simulink model "sysgenDWT"  (Simulink 7.0)
settings: Solver=ode45  StartTime=0.0  StopTime=4096+1024+100  RelTol=1e-3
PreLoadFcn:
  | xlrequire('imageData.mat'); xlrequire('PreLoadFcn');
PostLoadFcn:
  | open_system('sysgenDWT/Processor/Memory Controller','force'); pause(0.50); open_system('sysgenDWT');pause(0.50); close_system('sysgenDWT/Processor/Memory Controller');pause(0.50); close_system('sysgenDWT/Processor');
StopFcn:
  | xlrequire('StopFcn');
values from neighbouring files (symbols this model uses):
  b1Init = sysgenDWT_imageData( stride + dither )    [sysgenDWT_PreLoadFcn.m]
  b2Init = sysgenDWT_imageData( stride + not(dither) )    [sysgenDWT_PreLoadFcn.m]
libraries: xbsIndex_r4 x214, dspindex x4, dspmtrx3 x4, dspsnks4 x3, xbsCopyrightNotice_r4 x1, dspsrcs4 x1
(part 2 of 3)

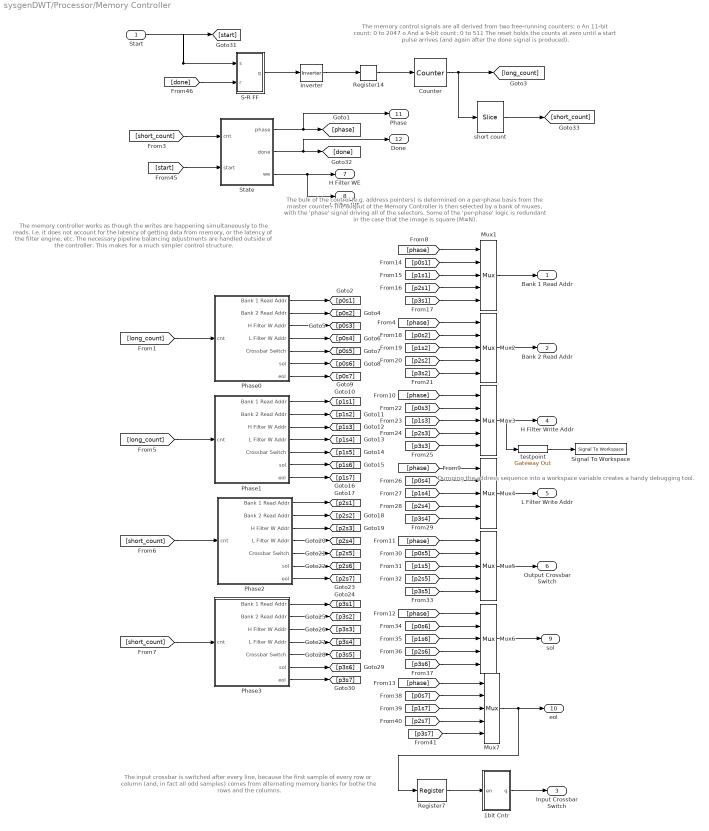
== system sysgenDWT/Processor/Memory Controller ==
  note: The memory control signals are all
      | derived from two free-running counters:
      |   o  An 11-bit count:    0 to 2047
      |   o  And a 9-bit count: 0 to 511
      | The reset holds the counts at zero until
      | a start pulse arrives (and again after the
      | done signal is produced).
  note: The bulk of the control (e.g. address pointers) is determined
      | on a per-phase basis from the master counter.  The output of
      | the Memory Controller is then selected by a bank of muxes,
      | with the 'phase' signal driving all of the selectors.  Some of
      | the 'per-phase' logic is redundant in the case that the image
      | is square (M=N).
  note: The memory controller works as though the
      | writes are happening simultaneously to the
      | reads. I.e. it does not account for the latency
      | of getting data from memory, or the latency
      | of the filter engine, etc.  The necessary
      | pipeline balancing adjustments are handled
      | outside of the controller.  This makes for a
      | much simpler control structure.
  note: The input crossbar is switched after every
      | line, because the first sample of every
      | row or column (and, in fact all odd samples)
      | comes from alternating memory banks for
      | bothe the rows and the columns.
  note: Dumping the address sequence
      | into a workspace variable creates
      | a handy debugging tool.
  Start : Inport  OutDataType=sfix(16)  OutScaling=2^0
  1bit Cntr : Subsystem
  Counter : xbsIndex_r4/Counter  cnt_type=Free Running  cnt_to=Inf  operation=Up  start_count=0  cnt_by_val=1  arith_type=Unsigned  n_bits=N+M-1  bin_pt=0  load_pin=off  rst=on  en=off  explicit_period=off  period=1  dbl_ovrd=off  use_behavioral_HDL=off  use_rpm=off  implementation=Fabric  block_type=counter
      settings: infoedit="Configurable up, down and up/down counter.<P><P>Hardware notes: Free running counters are the least expensive in hardware.  A count limited counter is implemented by combining a counter with a comparator."  xl_area=[6 11 0 11 0 0 0]  block_version=VER_STRING_GOES_HERE
  Inverter : xbsIndex_r4/Inverter  en=off  latency=0  dbl_ovrd=off  block_type=inv
      settings: xl_area=[1 0 0 1 0 0 0]  block_version=VER_STRING_GOES_HERE
  Mux{1..7} (7 alike) : xbsIndex_r4/Mux  inputs=4  en=off  latency=1  precision=Full  arith_type="Signed  (2's comp)"  n_bits=8  bin_pt=2  quantization=Truncate  overflow=Wrap  dbl_ovrd=off  block_type=mux
      Mux1 settings: xl_area=[11 11 0 22 0 0 0]  block_version=VER_STRING_GOES_HERE
      Mux2 settings: xl_area=[11 11 0 22 0 0 0]  block_version=VER_STRING_GOES_HERE
      Mux3 settings: xl_area=[11 11 0 22 0 0 0]  block_version=VER_STRING_GOES_HERE
      Mux4 settings: xl_area=[11 11 0 22 0 0 0]  block_version=VER_STRING_GOES_HERE
      Mux5 settings: xl_area=[1 1 0 2 0 0 0]  block_version=VER_STRING_GOES_HERE
      Mux6 settings: xl_area=[1 1 0 2 0 0 0]  block_version=VER_STRING_GOES_HERE
      Mux7 settings: xl_area=[1 1 0 2 0 0 0]  block_version=VER_STRING_GOES_HERE
  Phase0 : Subsystem
  Phase1 : Subsystem
  Phase2 : Subsystem
  Phase3 : Subsystem
  Register14 : xbsIndex_r4/Register  init=1  rst=off  en=off  dbl_ovrd=off  block_type=register
      settings: xl_area=[1 1 0 0 0 0 0]  block_version=VER_STRING_GOES_HERE
  Register7 : xbsIndex_r4/Register  init=0  rst=off  en=off  dbl_ovrd=off  block_type=register
      settings: xl_area=[1 1 0 0 0 0 0]  block_version=VER_STRING_GOES_HERE
  S-R FF : Subsystem
  Signal To Workspace : dspsnks4/Signal To Workspace  SystemSampleTime=-1  VariableName=HWriteAddr  FrameMode=Concatenate frames (2-D array)
      settings: FixptAsFi=off
  State : Subsystem
  short count : xbsIndex_r4/Slice  nbits=M+N-3  boolean_output=off  mode=Lower Bit Location + Width  bit1=0  base1=MSB of Input  bit0=0  base0=LSB of Input  dbl_ovrd=off  block_type=slice
      settings: infoedit="Extracts a given range of bits from each input sample and presents it at the output.  The output type is ordinarily unsigned with binary point at zero, but can be Boolean when the slice is one bit wide.<P><P>Hardware notes: In hardware this block costs nothing."  block_version=VER_STRING_GOES_HERE
  testpoint : xbsIndex_r4/Gateway Out  hdl_port=off  timing_constraint=None  locs_specified=off  LOCs={}  block_type=gatewayout
      settings: infoedit="Gateway out block.  Converts Xilinx fixed point inputs into ouputs of type Simulink integer, double, or fixed point.<P><P>Hardware notes:  In hardware these blocks become top level output ports or are discarded, depending on how they are configured."  xl_area=[0 0 0 0 0 0 0]  block_version=VER_STRING_GOES_HERE
  Bank 1 Read Addr : Outport  OutDataType=sfix(16)  OutScaling=2^0
  Bank 2 Read Addr : Outport  Port=2  OutDataType=sfix(16)  OutScaling=2^0
  Input Crossbar Switch : Outport  Port=3  OutDataType=sfix(16)  OutScaling=2^0
  H Filter Write Addr : Outport  Port=4  OutDataType=sfix(16)  OutScaling=2^0
  L Filter Write Addr : Outport  Port=5  OutDataType=sfix(16)  OutScaling=2^0
  Output Crossbar Switch : Outport  Port=6  OutDataType=sfix(16)  OutScaling=2^0
  H Filter WE : Outport  Port=7  OutDataType=sfix(16)  OutScaling=2^0
  L Filter WE : Outport  Port=8  OutDataType=sfix(16)  OutScaling=2^0
  sol : Outport  Port=9  OutDataType=sfix(16)  OutScaling=2^0
  eol : Outport  Port=10  OutDataType=sfix(16)  OutScaling=2^0
  Phase : Outport  Port=11  OutDataType=sfix(16)  OutScaling=2^0
  Done : Outport  Port=12  OutDataType=sfix(16)  OutScaling=2^0
  wires:
  Counter/1 -> [long_count], short count/1
  [long_count] -> Phase0/1(cnt)
  State/1(phase) -> Phase/1, [phase]
  [long_count] -> Phase1/1(cnt)
  [short_count] -> Phase2/1(cnt)
  [short_count] -> Phase3/1(cnt)
  [phase] -> Mux1/1
  [phase] -> Mux2/1
  [phase] -> Mux3/1
  [phase] -> Mux4/1
  [phase] -> Mux5/1
  [phase] -> Mux6/1
  [phase] -> Mux7/1
  Phase0/1(Bank 1 Read Addr) -> [p0s1]
  Phase0/2(Bank 2 Read Addr) -> [p0s2]
  Phase0/3(H Filter W Addr) -> [p0s3]
  Phase0/4(L Filter W Addr) -> [p0s4]
  Phase0/5(Crossbar Switch) -> [p0s5]
  Phase0/6(sol) -> [p0s6]
  Phase0/7(eol) -> [p0s7]
  Phase1/1(Bank 1 Read Addr) -> [p1s1]
  Phase1/2(Bank 2 Read Addr) -> [p1s2]
  Phase1/3(H Filter W Addr) -> [p1s3]
  Phase1/4(L Filter W Addr) -> [p1s4]
  Phase1/5(Crossbar Switch) -> [p1s5]
  Phase1/6(sol) -> [p1s6]
  Phase1/7(eol) -> [p1s7]
  Phase2/1(Bank 1 Read Addr) -> [p2s1]
  Phase2/2(Bank 2 Read Addr) -> [p2s2]
  Phase2/3(H Filter W Addr) -> [p2s3]
  Phase2/4(L Filter W Addr) -> [p2s4]
  Phase2/5(Crossbar Switch) -> [p2s5]
  Phase2/6(sol) -> [p2s6]
  Phase2/7(eol) -> [p2s7]
  Phase3/1(Bank 1 Read Addr) -> [p3s1]
  Phase3/2(Bank 2 Read Addr) -> [p3s2]
  Phase3/3(H Filter W Addr) -> [p3s3]
  Phase3/4(L Filter W Addr) -> [p3s4]
  Phase3/5(Crossbar Switch) -> [p3s5]
  Phase3/6(sol) -> [p3s6]
  Phase3/7(eol) -> [p3s7]
  [p0s1] -> Mux1/2
  [p1s1] -> Mux1/3
  [p2s1] -> Mux1/4
  [p3s1] -> Mux1/5
  [p0s2] -> Mux2/2
  [p1s2] -> Mux2/3
  [p2s2] -> Mux2/4
  [p3s2] -> Mux2/5
  [p0s3] -> Mux3/2
  [p1s3] -> Mux3/3
  [p2s3] -> Mux3/4
  [p3s3] -> Mux3/5
  [p0s4] -> Mux4/2
  [p1s4] -> Mux4/3
  [p2s4] -> Mux4/4
  [p3s4] -> Mux4/5
  [p0s5] -> Mux5/2
  [p1s5] -> Mux5/3
  [p2s5] -> Mux5/4
  [p3s5] -> Mux5/5
  [p0s6] -> Mux6/2
  [p1s6] -> Mux6/3
  [p2s6] -> Mux6/4
  [p3s6] -> Mux6/5
  [p0s7] -> Mux7/2
  [p1s7] -> Mux7/3
  [p2s7] -> Mux7/4
  [p3s7] -> Mux7/5
  Mux7/1 -> eol/1, Register7/1
  Mux6/1 -> sol/1
  Mux5/1 -> Output Crossbar Switch/1
  Mux4/1 -> L Filter Write Addr/1
  Mux3/1 -> H Filter Write Addr/1, testpoint/1
  Mux1/1 -> Bank 1 Read Addr/1
  Mux2/1 -> Bank 2 Read Addr/1
  1bit Cntr/1(q) -> Input Crossbar Switch/1
  Register7/1 -> 1bit Cntr/1(en)
  S-R FF/1(q) -> Inverter/1
  Start/1 -> S-R FF/1(s), [start]
  Register14/1 -> Counter/1
  Inverter/1 -> Register14/1
  [short_count] -> State/1(cnt)
  [start] -> State/2(start)
  State/3(we) -> L Filter WE/1, H Filter WE/1
  State/2(done) -> Done/1, [done]
  [done] -> S-R FF/2(r)
  short count/1 -> [short_count]
  testpoint/1 -> Signal To Workspace/1

== system sysgenDWT/Processor/Read Addr Crossbar ==
  note: Connect either A to A' and B to B'
      | or A to B' and B to A' based on
      | the signal "Cross".
  A : Inport  OutDataType=sfix(16)  OutScaling=2^0
  B : Inport  Port=2  OutDataType=sfix(16)  OutScaling=2^0
  Cross : Inport  Port=3  OutDataType=sfix(16)  OutScaling=2^0
  Mux2 : xbsIndex_r4/Mux  inputs=2  en=off  latency=0  precision=Full  arith_type="Signed  (2's comp)"  n_bits=8  bin_pt=2  quantization=Truncate  overflow=Wrap  dbl_ovrd=off  block_type=mux
      settings: xl_area=[6 0 0 11 0 0 0]  block_version=VER_STRING_GOES_HERE
  Mux3 : xbsIndex_r4/Mux  inputs=2  en=off  latency=0  precision=Full  arith_type="Signed  (2's comp)"  n_bits=8  bin_pt=2  quantization=Truncate  overflow=Wrap  dbl_ovrd=off  block_type=mux
      settings: xl_area=[6 0 0 11 0 0 0]  block_version=VER_STRING_GOES_HERE
  A' : Outport  OutDataType=sfix(16)  OutScaling=2^0
  B' : Outport  Port=2  OutDataType=sfix(16)  OutScaling=2^0
  wires:
  Cross/1 -> Mux3/1, Mux2/1
  B/1 -> Mux2/3, Mux3/2
  A/1 -> Mux3/3, Mux2/2
  Mux3/1 -> B'/1
  Mux2/1 -> A'/1

== system sysgenDWT/Processor/WE Crossbar ==
  note: Connect either A to A' and B to B'
      | or A to B' and B to A' based on
      | the signal "Cross".
  A : Inport  OutDataType=sfix(16)  OutScaling=2^0
  B : Inport  Port=2  OutDataType=sfix(16)  OutScaling=2^0
  Cross : Inport  Port=3  OutDataType=sfix(16)  OutScaling=2^0
  Mux2 : xbsIndex_r4/Mux  inputs=2  en=off  latency=1  precision=Full  arith_type="Signed  (2's comp)"  n_bits=8  bin_pt=2  quantization=Truncate  overflow=Wrap  dbl_ovrd=off  block_type=mux
      settings: xl_area=[1 1 0 1 0 0 0]  block_version=VER_STRING_GOES_HERE
  Mux3 : xbsIndex_r4/Mux  inputs=2  en=off  latency=1  precision=Full  arith_type="Signed  (2's comp)"  n_bits=8  bin_pt=2  quantization=Truncate  overflow=Wrap  dbl_ovrd=off  block_type=mux
      settings: xl_area=[1 1 0 1 0 0 0]  block_version=VER_STRING_GOES_HERE
  A' : Outport  OutDataType=sfix(16)  OutScaling=2^0
  B' : Outport  Port=2  OutDataType=sfix(16)  OutScaling=2^0
  wires:
  Mux2/1 -> A'/1
  Mux3/1 -> B'/1
  A/1 -> Mux2/2, Mux3/3
  B/1 -> Mux3/2, Mux2/3
  Cross/1 -> Mux2/1, Mux3/1

== system sysgenDWT/Processor/Write Addr Crossbar ==
  note: Connect either A to A' and B to B'
      | or A to B' and B to A' based on
      | the signal "Cross".
  A : Inport  OutDataType=sfix(16)  OutScaling=2^0
  B : Inport  Port=2  OutDataType=sfix(16)  OutScaling=2^0
  Cross : Inport  Port=3  OutDataType=sfix(16)  OutScaling=2^0
  Mux2 : xbsIndex_r4/Mux  inputs=2  en=off  latency=1  precision=Full  arith_type="Signed  (2's comp)"  n_bits=8  bin_pt=2  quantization=Truncate  overflow=Wrap  dbl_ovrd=off  block_type=mux
      settings: xl_area=[6 11 0 11 0 0 0]  block_version=VER_STRING_GOES_HERE
  Mux3 : xbsIndex_r4/Mux  inputs=2  en=off  latency=1  precision=Full  arith_type="Signed  (2's comp)"  n_bits=8  bin_pt=2  quantization=Truncate  overflow=Wrap  dbl_ovrd=off  block_type=mux
      settings: xl_area=[6 11 0 11 0 0 0]  block_version=VER_STRING_GOES_HERE
  A' : Outport  OutDataType=sfix(16)  OutScaling=2^0
  B' : Outport  Port=2  OutDataType=sfix(16)  OutScaling=2^0
  wires:
  Mux2/1 -> A'/1
  Mux3/1 -> B'/1
  A/1 -> Mux2/2, Mux3/3
  B/1 -> Mux3/2, Mux2/3
  Cross/1 -> Mux2/1, Mux3/1

== system sysgenDWT/Processor/Memory Controller/1bit Cntr ==
  note: A 1-bit, synchronous counter.
      |
      | The Convert block does no work, it
      | just gives simulink a hint as to what
      | the feedback type is.
  en : Inport  OutDataType=sfix(16)  OutScaling=2^0
  Convert : xbsIndex_r4/Convert  Orientation=left  arith_type=Unsigned  n_bits=1  bin_pt=0  quantization=Truncate  overflow=Wrap  latency=0  dbl_ovrd=off  pipeline=off  block_type=convert
      settings: infoedit=The input is presented at the output after quantization and overflow effects.<P><P>Hardware notes: Additional hardware is used when rounding or saturation is selected and output width is less than the input width.  xl_area=[0 0 0 0 0 0 0]  block_version=VER_STRING_GOES_HERE
  Inverter1 : xbsIndex_r4/Inverter  en=off  latency=0  dbl_ovrd=off  block_type=inv
      settings: xl_area=[1 0 0 1 0 0 0]  block_version=VER_STRING_GOES_HERE
  Register6 : xbsIndex_r4/Register  init=1  rst=off  en=on  dbl_ovrd=off  block_type=register
      settings: xl_area=[1 1 0 0 0 0 0]  block_version=VER_STRING_GOES_HERE
  q : Outport  OutDataType=sfix(16)  OutScaling=2^0
  wires:
  Inverter1/1 -> Register6/1
  Register6/1 -> Convert/1, q/1
  Convert/1 -> Inverter1/1
  en/1 -> Register6/2

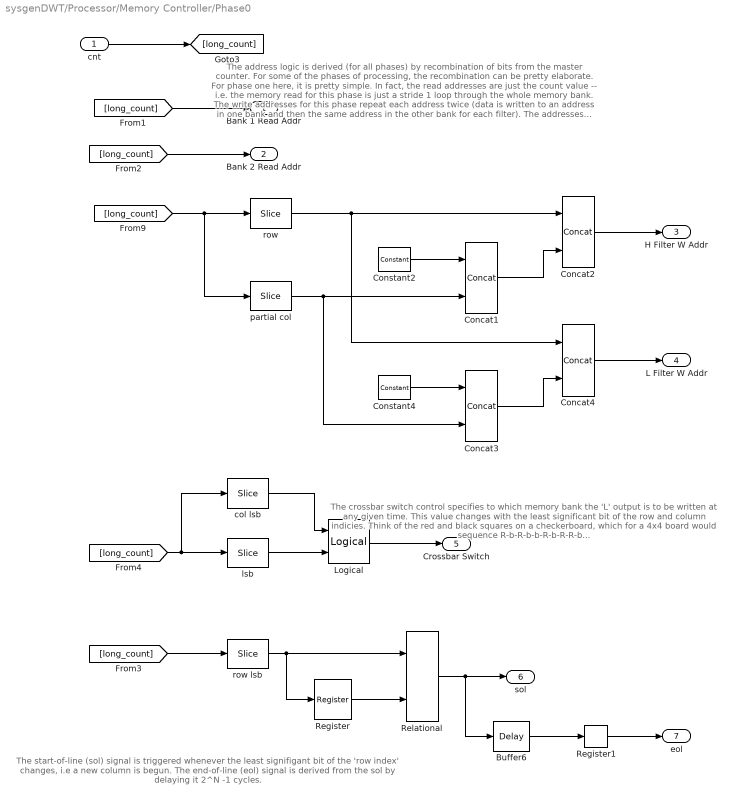
== system sysgenDWT/Processor/Memory Controller/Phase0 ==
  note: The address logic is derived (for all phases) by recombination
      | of bits from the master counter. For some of the phases of
      | processing, the recombination can be pretty elaborate.  For
      | phase one here, it is pretty simple.  In fact, the read addresses
      | are just the count value -- i.e. the memory read for this phase
      | is just a stride 1 loop through the whole memory bank.  The
      | write addresses for this phase repeat each address twice (data
      | is written to an address in one bank and then the same address
      | in the other bank for each filter).  The addresses increment by
      | one as each column is processed, and then jump to the next
      | column. A '1' is injected into the H address and a '0' into the 'L'
      | adress to write to the lower or upper half of memory, respectively.
  note: The crossbar switch control specifies to which memory
      | bank the 'L' output is to be written at any given time.
      | This value changes with the least significant bit of the
      | row and column indicies.  Think of the red and black
      | squares on a checkerboard, which for a 4x4 board would
      | sequence R-b-R-b-b-R-b-R-R-b...
  note: The start-of-line (sol) signal is triggered whenever the
      | least signifigant bit of the 'row index' changes, i.e a
      | new column is begun.  The end-of-line (eol) signal is
      | derived from the sol by delaying it 2^N -1 cycles.
  cnt : Inport  OutDataType=sfix(16)  OutScaling=2^0
  Buffer6 : xbsIndex_r4/Delay  en=off  latency=power(2,N-1)-2  dbl_ovrd=off  reg_retiming=off  block_type=delay
      settings: infoedit="Delay line having  configurable length.<P><P>Hardware notes: A delay line is a chain, each link of which is an SRL16 followed by a flip-flop. If register retiming is enabled, the delay line is a chain of flip-flops."  xl_area=[2 2 0 2 0 0 0]  block_version=VER_STRING_GOES_HERE
  Concat{1..4} (4 alike) : xbsIndex_r4/Concat  num_inputs=2  dbl_ovrd=off  block_type=concat
      settings: block_version=VER_STRING_GOES_HERE
  Constant2 : xbsIndex_r4/Constant  arith_type=Unsigned  const=1  n_bits=1  bin_pt=0  explicit_period=off  period=1  equ=P=C  opselect=C  inp2=PCIN>>17  opr=+  inp1=P  carry=CIN  dbl_ovrd=off  block_type=constant
      settings: block_version=VER_STRING_GOES_HERE
  Constant4 : xbsIndex_r4/Constant  arith_type=Unsigned  const=0  n_bits=1  bin_pt=0  explicit_period=off  period=1  equ=P=C  opselect=C  inp2=PCIN>>17  opr=+  inp1=P  carry=CIN  dbl_ovrd=off  block_type=constant
      settings: block_version=VER_STRING_GOES_HERE
  Logical : xbsIndex_r4/Logical  logical_function=XNOR  inputs=2  en=off  latency=0  precision=Full  arith_type=Unsigned  n_bits=8  bin_pt=2  align_bp=on  dbl_ovrd=off  block_type=logical
      settings: xl_area=[1 0 0 1 0 0 0]  block_version=VER_STRING_GOES_HERE
  Register : xbsIndex_r4/Register  init=1  rst=off  en=off  dbl_ovrd=off  block_type=register
      settings: xl_area=[1 1 0 0 0 0 0]  block_version=VER_STRING_GOES_HERE
  Register1 : xbsIndex_r4/Register  init=0  rst=off  en=off  dbl_ovrd=off  block_type=register
      settings: xl_area=[1 1 0 0 0 0 0]  block_version=VER_STRING_GOES_HERE
  Relational : xbsIndex_r4/Relational  mode=a!=b  en=off  latency=0  dbl_ovrd=off  block_type=relational
      settings: xl_area=[1 0 0 1 0 0 0]  block_version=VER_STRING_GOES_HERE
  col lsb : xbsIndex_r4/Slice  nbits=1  boolean_output=off  mode=Lower Bit Location + Width  bit1=0  base1=MSB of Input  bit0=M-1  base0=LSB of Input  dbl_ovrd=off  block_type=slice
      settings: infoedit="Extracts a given range of bits from each input sample and presents it at the output.  The output type is ordinarily unsigned with binary point at zero, but can be Boolean when the slice is one bit wide.<P><P>Hardware notes: In hardware this block costs nothing."  block_version=VER_STRING_GOES_HERE
  lsb : xbsIndex_r4/Slice  nbits=1  boolean_output=off  mode=Lower Bit Location + Width  bit1=0  base1=MSB of Input  bit0=0  base0=LSB of Input  dbl_ovrd=off  block_type=slice
      settings: infoedit="Extracts a given range of bits from each input sample and presents it at the output.  The output type is ordinarily unsigned with binary point at zero, but can be Boolean when the slice is one bit wide.<P><P>Hardware notes: In hardware this block costs nothing."  block_version=VER_STRING_GOES_HERE
  partial col : xbsIndex_r4/Slice  nbits=N-2  boolean_output=off  mode=Lower Bit Location + Width  bit1=0  base1=MSB of Input  bit0=1  base0=LSB of Input  dbl_ovrd=off  block_type=slice
      settings: infoedit="Extracts a given range of bits from each input sample and presents it at the output.  The output type is ordinarily unsigned with binary point at zero, but can be Boolean when the slice is one bit wide.<P><P>Hardware notes: In hardware this block costs nothing."  block_version=VER_STRING_GOES_HERE
  row : xbsIndex_r4/Slice  nbits=M  boolean_output=off  mode=Upper Bit Location + Width  bit1=0  base1=MSB of Input  bit0=N  base0=LSB of Input  dbl_ovrd=off  block_type=slice
      settings: infoedit="Extracts a given range of bits from each input sample and presents it at the output.  The output type is ordinarily unsigned with binary point at zero, but can be Boolean when the slice is one bit wide.<P><P>Hardware notes: In hardware this block costs nothing."  block_version=VER_STRING_GOES_HERE
  row lsb : xbsIndex_r4/Slice  nbits=1  boolean_output=off  mode=Lower Bit Location + Width  bit1=0  base1=MSB of Input  bit0=N-1  base0=LSB of Input  dbl_ovrd=off  block_type=slice
      settings: infoedit="Extracts a given range of bits from each input sample and presents it at the output.  The output type is ordinarily unsigned with binary point at zero, but can be Boolean when the slice is one bit wide.<P><P>Hardware notes: In hardware this block costs nothing."  block_version=VER_STRING_GOES_HERE
  Bank 1 Read Addr : Outport  OutDataType=sfix(16)  OutScaling=2^0
  Bank 2 Read Addr : Outport  Port=2  OutDataType=sfix(16)  OutScaling=2^0
  H Filter W Addr : Outport  Port=3  OutDataType=sfix(16)  OutScaling=2^0
  L Filter W Addr : Outport  Port=4  OutDataType=sfix(16)  OutScaling=2^0
  Crossbar Switch : Outport  Port=5  OutDataType=sfix(16)  OutScaling=2^0
  sol : Outport  Port=6  OutDataType=sfix(16)  OutScaling=2^0
  eol : Outport  Port=7  OutDataType=sfix(16)  OutScaling=2^0
  wires:
  [long_count] -> Bank 2 Read Addr/1
  [long_count] -> row lsb/1
  row lsb/1 -> Relational/1, Register/1
  Relational/1 -> sol/1, Buffer6/1
  Buffer6/1 -> Register1/1
  [long_count] -> lsb/1, col lsb/1
  Register/1 -> Relational/2
  [long_count] -> row/1, partial col/1
  row/1 -> Concat4/1, Concat2/1
  Constant2/1 -> Concat1/1
  Constant4/1 -> Concat3/1
  Concat3/1 -> Concat4/2
  partial col/1 -> Concat3/2, Concat1/2
  Concat1/1 -> Concat2/2
  [long_count] -> Bank 1 Read Addr/1
  Concat2/1 -> H Filter W Addr/1
  Concat4/1 -> L Filter W Addr/1
  Register1/1 -> eol/1
  cnt/1 -> [long_count]
  lsb/1 -> Logical/2
  col lsb/1 -> Logical/1
  Logical/1 -> Crossbar Switch/1

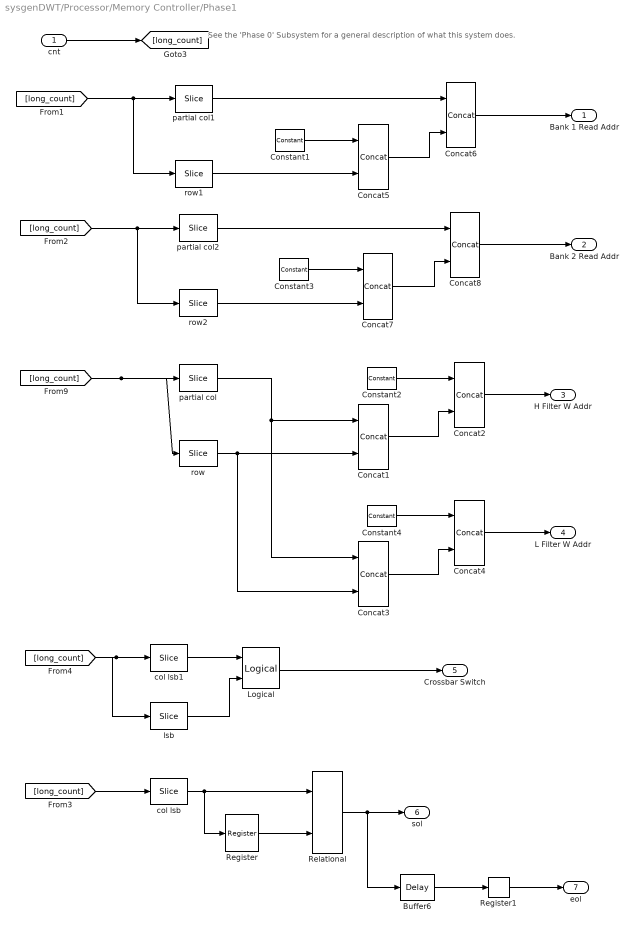
== system sysgenDWT/Processor/Memory Controller/Phase1 ==
  note: See the 'Phase 0' Subsystem for a general
      | description of what this system does.
  cnt : Inport  OutDataType=sfix(16)  OutScaling=2^0
  Buffer6 : xbsIndex_r4/Delay  en=off  latency=power(2,N-1)-2  dbl_ovrd=off  reg_retiming=off  block_type=delay
      settings: infoedit="Delay line having  configurable length.<P><P>Hardware notes: A delay line is a chain, each link of which is an SRL16 followed by a flip-flop. If register retiming is enabled, the delay line is a chain of flip-flops."  xl_area=[2 2 0 2 0 0 0]  block_version=VER_STRING_GOES_HERE
  Concat{1..8} (8 alike) : xbsIndex_r4/Concat  num_inputs=2  dbl_ovrd=off  block_type=concat
      settings: block_version=VER_STRING_GOES_HERE
  Constant1 : xbsIndex_r4/Constant  arith_type=Unsigned  const=1  n_bits=1  bin_pt=0  explicit_period=off  period=1  equ=P=C  opselect=C  inp2=PCIN>>17  opr=+  inp1=P  carry=CIN  dbl_ovrd=off  block_type=constant
      settings: block_version=VER_STRING_GOES_HERE
  Constant2 : xbsIndex_r4/Constant  arith_type=Unsigned  const=1  n_bits=1  bin_pt=0  explicit_period=off  period=1  equ=P=C  opselect=C  inp2=PCIN>>17  opr=+  inp1=P  carry=CIN  dbl_ovrd=off  block_type=constant
      settings: block_version=VER_STRING_GOES_HERE
  Constant3 : xbsIndex_r4/Constant  arith_type=Unsigned  const=0  n_bits=1  bin_pt=0  explicit_period=off  period=1  equ=P=C  opselect=C  inp2=PCIN>>17  opr=+  inp1=P  carry=CIN  dbl_ovrd=off  block_type=constant
      settings: block_version=VER_STRING_GOES_HERE
  Constant4 : xbsIndex_r4/Constant  arith_type=Unsigned  const=0  n_bits=1  bin_pt=0  explicit_period=off  period=1  equ=P=C  opselect=C  inp2=PCIN>>17  opr=+  inp1=P  carry=CIN  dbl_ovrd=off  block_type=constant
      settings: block_version=VER_STRING_GOES_HERE
  Logical : xbsIndex_r4/Logical  logical_function=XNOR  inputs=2  en=off  latency=0  precision=Full  arith_type=Unsigned  n_bits=8  bin_pt=2  align_bp=on  dbl_ovrd=off  block_type=logical
      settings: xl_area=[1 0 0 1 0 0 0]  block_version=VER_STRING_GOES_HERE
  Register : xbsIndex_r4/Register  init=1  rst=off  en=off  dbl_ovrd=off  block_type=register
      settings: xl_area=[1 1 0 0 0 0 0]  block_version=VER_STRING_GOES_HERE
  Register1 : xbsIndex_r4/Register  init=0  rst=off  en=off  dbl_ovrd=off  block_type=register
      settings: xl_area=[1 1 0 0 0 0 0]  block_version=VER_STRING_GOES_HERE
  Relational : xbsIndex_r4/Relational  mode=a!=b  en=off  latency=0  dbl_ovrd=off  block_type=relational
      settings: xl_area=[1 0 0 1 0 0 0]  block_version=VER_STRING_GOES_HERE
  col lsb : xbsIndex_r4/Slice  nbits=1  boolean_output=off  mode=Lower Bit Location + Width  bit1=0  base1=MSB of Input  bit0=M-1  base0=LSB of Input  dbl_ovrd=off  block_type=slice
      settings: infoedit="Extracts a given range of bits from each input sample and presents it at the output.  The output type is ordinarily unsigned with binary point at zero, but can be Boolean when the slice is one bit wide.<P><P>Hardware notes: In hardware this block costs nothing."  block_version=VER_STRING_GOES_HERE
  col lsb1 : xbsIndex_r4/Slice  nbits=1  boolean_output=off  mode=Lower Bit Location + Width  bit1=0  base1=MSB of Input  bit0=M-1  base0=LSB of Input  dbl_ovrd=off  block_type=slice
      settings: infoedit="Extracts a given range of bits from each input sample and presents it at the output.  The output type is ordinarily unsigned with binary point at zero, but can be Boolean when the slice is one bit wide.<P><P>Hardware notes: In hardware this block costs nothing."  block_version=VER_STRING_GOES_HERE
  lsb : xbsIndex_r4/Slice  nbits=1  boolean_output=off  mode=Lower Bit Location + Width  bit1=0  base1=MSB of Input  bit0=0  base0=LSB of Input  dbl_ovrd=off  block_type=slice
      settings: infoedit="Extracts a given range of bits from each input sample and presents it at the output.  The output type is ordinarily unsigned with binary point at zero, but can be Boolean when the slice is one bit wide.<P><P>Hardware notes: In hardware this block costs nothing."  block_version=VER_STRING_GOES_HERE
  partial col : xbsIndex_r4/Slice  nbits=N-1  boolean_output=off  mode=Lower Bit Location + Width  bit1=0  base1=MSB of Input  bit0=0  base0=LSB of Input  dbl_ovrd=off  block_type=slice
      settings: infoedit="Extracts a given range of bits from each input sample and presents it at the output.  The output type is ordinarily unsigned with binary point at zero, but can be Boolean when the slice is one bit wide.<P><P>Hardware notes: In hardware this block costs nothing."  block_version=VER_STRING_GOES_HERE
  partial col1 : xbsIndex_r4/Slice  nbits=N-1  boolean_output=off  mode=Lower Bit Location + Width  bit1=0  base1=MSB of Input  bit0=0  base0=LSB of Input  dbl_ovrd=off  block_type=slice
      settings: infoedit="Extracts a given range of bits from each input sample and presents it at the output.  The output type is ordinarily unsigned with binary point at zero, but can be Boolean when the slice is one bit wide.<P><P>Hardware notes: In hardware this block costs nothing."  block_version=VER_STRING_GOES_HERE
  partial col2 : xbsIndex_r4/Slice  nbits=N-1  boolean_output=off  mode=Lower Bit Location + Width  bit1=0  base1=MSB of Input  bit0=0  base0=LSB of Input  dbl_ovrd=off  block_type=slice
      settings: infoedit="Extracts a given range of bits from each input sample and presents it at the output.  The output type is ordinarily unsigned with binary point at zero, but can be Boolean when the slice is one bit wide.<P><P>Hardware notes: In hardware this block costs nothing."  block_version=VER_STRING_GOES_HERE
  row : xbsIndex_r4/Slice  nbits=M-1  boolean_output=off  mode=Upper Bit Location + Width  bit1=0  base1=MSB of Input  bit0=N  base0=LSB of Input  dbl_ovrd=off  block_type=slice
      settings: infoedit="Extracts a given range of bits from each input sample and presents it at the output.  The output type is ordinarily unsigned with binary point at zero, but can be Boolean when the slice is one bit wide.<P><P>Hardware notes: In hardware this block costs nothing."  block_version=VER_STRING_GOES_HERE
  row1 : xbsIndex_r4/Slice  nbits=M-1  boolean_output=off  mode=Upper Bit Location + Width  bit1=0  base1=MSB of Input  bit0=N  base0=LSB of Input  dbl_ovrd=off  block_type=slice
      settings: infoedit="Extracts a given range of bits from each input sample and presents it at the output.  The output type is ordinarily unsigned with binary point at zero, but can be Boolean when the slice is one bit wide.<P><P>Hardware notes: In hardware this block costs nothing."  block_version=VER_STRING_GOES_HERE
  row2 : xbsIndex_r4/Slice  nbits=M-1  boolean_output=off  mode=Upper Bit Location + Width  bit1=0  base1=MSB of Input  bit0=N  base0=LSB of Input  dbl_ovrd=off  block_type=slice
      settings: infoedit="Extracts a given range of bits from each input sample and presents it at the output.  The output type is ordinarily unsigned with binary point at zero, but can be Boolean when the slice is one bit wide.<P><P>Hardware notes: In hardware this block costs nothing."  block_version=VER_STRING_GOES_HERE
  Bank 1 Read Addr : Outport  OutDataType=sfix(16)  OutScaling=2^0
  Bank 2 Read Addr : Outport  Port=2  OutDataType=sfix(16)  OutScaling=2^0
  H Filter W Addr : Outport  Port=3  OutDataType=sfix(16)  OutScaling=2^0
  L Filter W Addr : Outport  Port=4  OutDataType=sfix(16)  OutScaling=2^0
  Crossbar Switch : Outport  Port=5  OutDataType=sfix(16)  OutScaling=2^0
  sol : Outport  Port=6  OutDataType=sfix(16)  OutScaling=2^0
  eol : Outport  Port=7  OutDataType=sfix(16)  OutScaling=2^0
  wires:
  cnt/1 -> [long_count]
  Register1/1 -> eol/1
  Concat4/1 -> L Filter W Addr/1
  Concat2/1 -> H Filter W Addr/1
  Concat1/1 -> Concat2/2
  Concat3/1 -> Concat4/2
  [long_count] -> partial col/1, row/1
  Register/1 -> Relational/2
  lsb/1 -> Logical/2
  [long_count] -> lsb/1, col lsb1/1
  Buffer6/1 -> Register1/1
  Relational/1 -> Buffer6/1, sol/1
  col lsb/1 -> Register/1, Relational/1
  [long_count] -> col lsb/1
  Concat5/1 -> Concat6/2
  partial col1/1 -> Concat6/1
  Concat6/1 -> Bank 1 Read Addr/1
  row1/1 -> Concat5/2
  [long_count] -> partial col1/1, row1/1
  Concat7/1 -> Concat8/2
  partial col2/1 -> Concat8/1
  Concat8/1 -> Bank 2 Read Addr/1
  row2/1 -> Concat7/2
  [long_count] -> partial col2/1, row2/1
  Constant2/1 -> Concat2/1
  Constant4/1 -> Concat4/1
  row/1 -> Concat1/2, Concat3/2
  Constant1/1 -> Concat5/1
  Constant3/1 -> Concat7/1
  col lsb1/1 -> Logical/1
  Logical/1 -> Crossbar Switch/1
  partial col/1 -> Concat1/1, Concat3/1

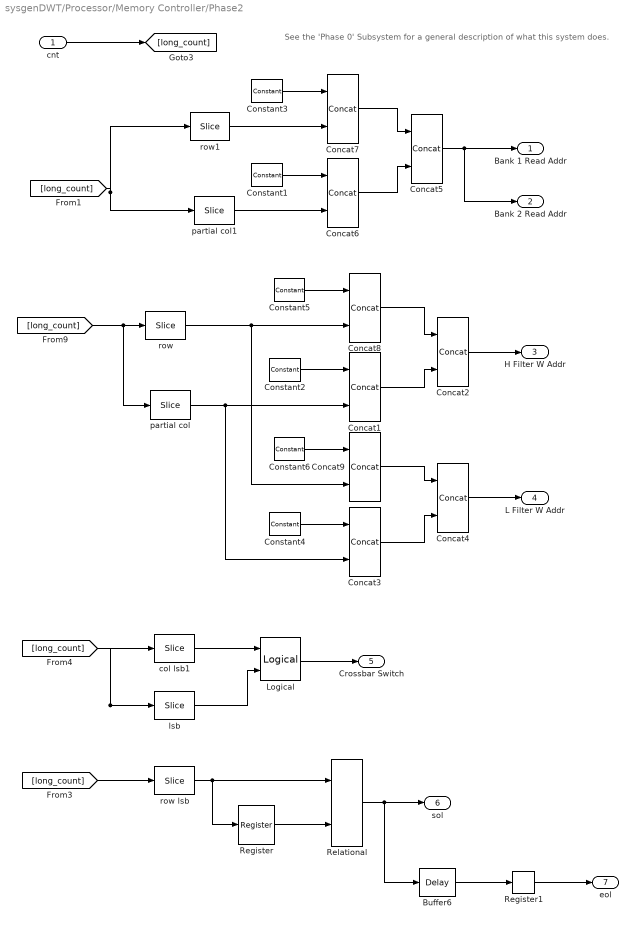
== system sysgenDWT/Processor/Memory Controller/Phase2 ==
  note: See the 'Phase 0' Subsystem for a general
      | description of what this system does.
  cnt : Inport  OutDataType=sfix(16)  OutScaling=2^0
  Buffer6 : xbsIndex_r4/Delay  en=off  latency=power(2,N-1)-2  dbl_ovrd=off  reg_retiming=off  block_type=delay
      settings: infoedit="Delay line having  configurable length.<P><P>Hardware notes: A delay line is a chain, each link of which is an SRL16 followed by a flip-flop. If register retiming is enabled, the delay line is a chain of flip-flops."  xl_area=[2 2 0 2 0 0 0]  block_version=VER_STRING_GOES_HERE
  Concat{1..9} (9 alike) : xbsIndex_r4/Concat  num_inputs=2  dbl_ovrd=off  block_type=concat
      settings: block_version=VER_STRING_GOES_HERE
  Constant{1,3,5..6} (4 alike) : xbsIndex_r4/Constant  arith_type=Unsigned  const=0  n_bits=1  bin_pt=0  explicit_period=off  period=1  equ=P=C  opselect=C  inp2=PCIN>>17  opr=+  inp1=P  carry=CIN  dbl_ovrd=off  block_type=constant
      settings: block_version=VER_STRING_GOES_HERE
  Constant2 : xbsIndex_r4/Constant  arith_type=Unsigned  const=1  n_bits=2  bin_pt=0  explicit_period=off  period=1  equ=P=C  opselect=C  inp2=PCIN>>17  opr=+  inp1=P  carry=CIN  dbl_ovrd=off  block_type=constant
      settings: block_version=VER_STRING_GOES_HERE
  Constant4 : xbsIndex_r4/Constant  arith_type=Unsigned  const=0  n_bits=2  bin_pt=0  explicit_period=off  period=1  equ=P=C  opselect=C  inp2=PCIN>>17  opr=+  inp1=P  carry=CIN  dbl_ovrd=off  block_type=constant
      settings: block_version=VER_STRING_GOES_HERE
  Logical : xbsIndex_r4/Logical  logical_function=XNOR  inputs=2  en=off  latency=0  precision=Full  arith_type=Unsigned  n_bits=8  bin_pt=2  align_bp=on  dbl_ovrd=off  block_type=logical
      settings: xl_area=[1 0 0 1 0 0 0]  block_version=VER_STRING_GOES_HERE
  Register : xbsIndex_r4/Register  init=1  rst=off  en=off  dbl_ovrd=off  block_type=register
      settings: xl_area=[1 1 0 0 0 0 0]  block_version=VER_STRING_GOES_HERE
  Register1 : xbsIndex_r4/Register  init=0  rst=off  en=off  dbl_ovrd=off  block_type=register
      settings: xl_area=[1 1 0 0 0 0 0]  block_version=VER_STRING_GOES_HERE
  Relational : xbsIndex_r4/Relational  mode=a!=b  en=off  latency=0  dbl_ovrd=off  block_type=relational
      settings: xl_area=[1 0 0 1 0 0 0]  block_version=VER_STRING_GOES_HERE
  col lsb1 : xbsIndex_r4/Slice  nbits=1  boolean_output=off  mode=Lower Bit Location + Width  bit1=0  base1=MSB of Input  bit0=N-2  base0=LSB of Input  dbl_ovrd=off  block_type=slice
      settings: infoedit="Extracts a given range of bits from each input sample and presents it at the output.  The output type is ordinarily unsigned with binary point at zero, but can be Boolean when the slice is one bit wide.<P><P>Hardware notes: In hardware this block costs nothing."  block_version=VER_STRING_GOES_HERE
  lsb : xbsIndex_r4/Slice  nbits=1  boolean_output=off  mode=Lower Bit Location + Width  bit1=0  base1=MSB of Input  bit0=0  base0=LSB of Input  dbl_ovrd=off  block_type=slice
      settings: infoedit="Extracts a given range of bits from each input sample and presents it at the output.  The output type is ordinarily unsigned with binary point at zero, but can be Boolean when the slice is one bit wide.<P><P>Hardware notes: In hardware this block costs nothing."  block_version=VER_STRING_GOES_HERE
  partial col : xbsIndex_r4/Slice  nbits=N-3  boolean_output=off  mode=Lower Bit Location + Width  bit1=0  base1=MSB of Input  bit0=1  base0=LSB of Input  dbl_ovrd=off  block_type=slice
      settings: infoedit="Extracts a given range of bits from each input sample and presents it at the output.  The output type is ordinarily unsigned with binary point at zero, but can be Boolean when the slice is one bit wide.<P><P>Hardware notes: In hardware this block costs nothing."  block_version=VER_STRING_GOES_HERE
  partial col1 : xbsIndex_r4/Slice  nbits=N-2  boolean_output=off  mode=Lower Bit Location + Width  bit1=0  base1=MSB of Input  bit0=0  base0=LSB of Input  dbl_ovrd=off  block_type=slice
      settings: infoedit="Extracts a given range of bits from each input sample and presents it at the output.  The output type is ordinarily unsigned with binary point at zero, but can be Boolean when the slice is one bit wide.<P><P>Hardware notes: In hardware this block costs nothing."  block_version=VER_STRING_GOES_HERE
  row : xbsIndex_r4/Slice  nbits=M-1  boolean_output=off  mode=Upper Bit Location + Width  bit1=0  base1=MSB of Input  bit0=N  base0=LSB of Input  dbl_ovrd=off  block_type=slice
      settings: infoedit="Extracts a given range of bits from each input sample and presents it at the output.  The output type is ordinarily unsigned with binary point at zero, but can be Boolean when the slice is one bit wide.<P><P>Hardware notes: In hardware this block costs nothing."  block_version=VER_STRING_GOES_HERE
  row lsb : xbsIndex_r4/Slice  nbits=1  boolean_output=off  mode=Lower Bit Location + Width  bit1=0  base1=MSB of Input  bit0=N-2  base0=LSB of Input  dbl_ovrd=off  block_type=slice
      settings: infoedit="Extracts a given range of bits from each input sample and presents it at the output.  The output type is ordinarily unsigned with binary point at zero, but can be Boolean when the slice is one bit wide.<P><P>Hardware notes: In hardware this block costs nothing."  block_version=VER_STRING_GOES_HERE
  row1 : xbsIndex_r4/Slice  nbits=M-1  boolean_output=off  mode=Upper Bit Location + Width  bit1=0  base1=MSB of Input  bit0=N  base0=LSB of Input  dbl_ovrd=off  block_type=slice
      settings: infoedit="Extracts a given range of bits from each input sample and presents it at the output.  The output type is ordinarily unsigned with binary point at zero, but can be Boolean when the slice is one bit wide.<P><P>Hardware notes: In hardware this block costs nothing."  block_version=VER_STRING_GOES_HERE
  Bank 1 Read Addr : Outport  OutDataType=sfix(16)  OutScaling=2^0
  Bank 2 Read Addr : Outport  Port=2  OutDataType=sfix(16)  OutScaling=2^0
  H Filter W Addr : Outport  Port=3  OutDataType=sfix(16)  OutScaling=2^0
  L Filter W Addr : Outport  Port=4  OutDataType=sfix(16)  OutScaling=2^0
  Crossbar Switch : Outport  Port=5  OutDataType=sfix(16)  OutScaling=2^0
  sol : Outport  Port=6  OutDataType=sfix(16)  OutScaling=2^0
  eol : Outport  Port=7  OutDataType=sfix(16)  OutScaling=2^0
  wires:
  Logical/1 -> Crossbar Switch/1
  col lsb1/1 -> Logical/1
  lsb/1 -> Logical/2
  cnt/1 -> [long_count]
  Register1/1 -> eol/1
  Concat4/1 -> L Filter W Addr/1
  Concat2/1 -> H Filter W Addr/1
  Concat1/1 -> Concat2/2
  partial col/1 -> Concat1/2, Concat3/2
  Concat3/1 -> Concat4/2
  Constant4/1 -> Concat3/1
  Constant2/1 -> Concat1/1
  row/1 -> Concat8/2, Concat9/2
  [long_count] -> partial col/1, row/1
  Register/1 -> Relational/2
  [long_count] -> col lsb1/1, lsb/1
  Buffer6/1 -> Register1/1
  Relational/1 -> Buffer6/1, sol/1
  row lsb/1 -> Register/1, Relational/1
  [long_count] -> row lsb/1
  Concat5/1 -> Bank 1 Read Addr/1, Bank 2 Read Addr/1
  Constant1/1 -> Concat6/1
  partial col1/1 -> Concat6/2
  [long_count] -> partial col1/1, row1/1
  Concat6/1 -> Concat5/2
  row1/1 -> Concat7/2
  Constant3/1 -> Concat7/1
  Concat7/1 -> Concat5/1
  Constant5/1 -> Concat8/1
  Concat8/1 -> Concat2/1
  Constant6/1 -> Concat9/1
  Concat9/1 -> Concat4/1

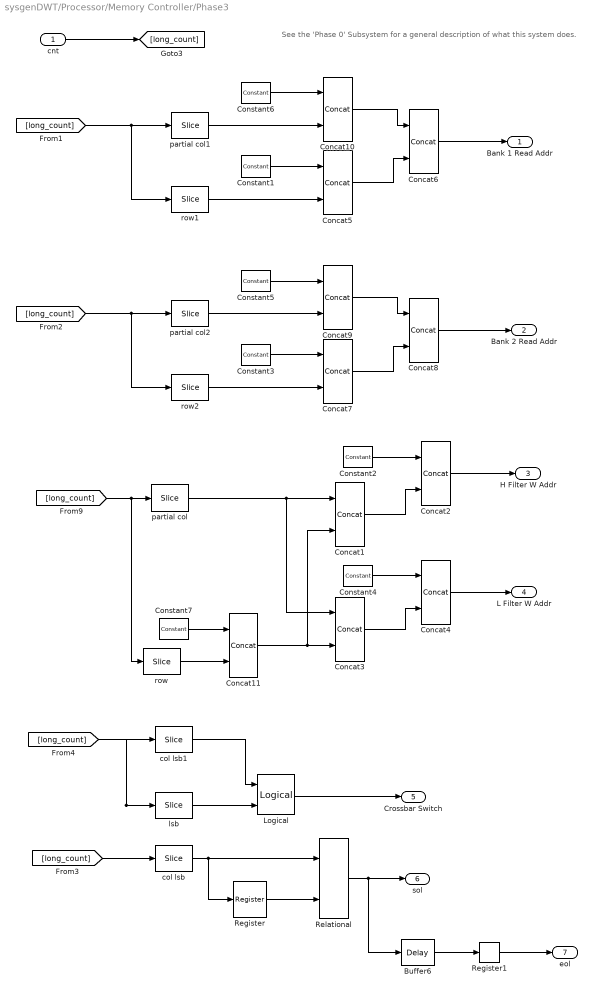
== system sysgenDWT/Processor/Memory Controller/Phase3 ==
  note: See the 'Phase 0' Subsystem for a general
      | description of what this system does.
  cnt : Inport  OutDataType=sfix(16)  OutScaling=2^0
  Buffer6 : xbsIndex_r4/Delay  en=off  latency=power(2,N-1)-2  dbl_ovrd=off  reg_retiming=off  block_type=delay
      settings: infoedit="Delay line having  configurable length.<P><P>Hardware notes: A delay line is a chain, each link of which is an SRL16 followed by a flip-flop. If register retiming is enabled, the delay line is a chain of flip-flops."  xl_area=[2 2 0 2 0 0 0]  block_version=VER_STRING_GOES_HERE
  Concat{1..11} (11 alike) : xbsIndex_r4/Concat  num_inputs=2  dbl_ovrd=off  block_type=concat
      settings: block_version=VER_STRING_GOES_HERE
  Constant1 : xbsIndex_r4/Constant  arith_type=Unsigned  const=2  n_bits=2  bin_pt=0  explicit_period=off  period=1  equ=P=C  opselect=C  inp2=PCIN>>17  opr=+  inp1=P  carry=CIN  dbl_ovrd=off  block_type=constant
      settings: block_version=VER_STRING_GOES_HERE
  Constant2 : xbsIndex_r4/Constant  arith_type=Unsigned  const=1  n_bits=2  bin_pt=0  explicit_period=off  period=1  equ=P=C  opselect=C  inp2=PCIN>>17  opr=+  inp1=P  carry=CIN  dbl_ovrd=off  block_type=constant
      settings: block_version=VER_STRING_GOES_HERE
  Constant3 : xbsIndex_r4/Constant  arith_type=Unsigned  const=0  n_bits=2  bin_pt=0  explicit_period=off  period=1  equ=P=C  opselect=C  inp2=PCIN>>17  opr=+  inp1=P  carry=CIN  dbl_ovrd=off  block_type=constant
      settings: block_version=VER_STRING_GOES_HERE
  Constant4 : xbsIndex_r4/Constant  arith_type=Unsigned  const=0  n_bits=2  bin_pt=0  explicit_period=off  period=1  equ=P=C  opselect=C  inp2=PCIN>>17  opr=+  inp1=P  carry=CIN  dbl_ovrd=off  block_type=constant
      settings: block_version=VER_STRING_GOES_HERE
  Constant5 : xbsIndex_r4/Constant  arith_type=Unsigned  const=0  n_bits=1  bin_pt=0  explicit_period=off  period=1  equ=P=C  opselect=C  inp2=PCIN>>17  opr=+  inp1=P  carry=CIN  dbl_ovrd=off  block_type=constant
      settings: block_version=VER_STRING_GOES_HERE
  Constant6 : xbsIndex_r4/Constant  arith_type=Unsigned  const=0  n_bits=1  bin_pt=0  explicit_period=off  period=1  equ=P=C  opselect=C  inp2=PCIN>>17  opr=+  inp1=P  carry=CIN  dbl_ovrd=off  block_type=constant
      settings: block_version=VER_STRING_GOES_HERE
  Constant7 : xbsIndex_r4/Constant  arith_type=Unsigned  const=0  n_bits=1  bin_pt=0  explicit_period=off  period=1  equ=P=C  opselect=C  inp2=PCIN>>17  opr=+  inp1=P  carry=CIN  dbl_ovrd=off  block_type=constant
      settings: block_version=VER_STRING_GOES_HERE
  Logical : xbsIndex_r4/Logical  logical_function=XNOR  inputs=2  en=off  latency=0  precision=Full  arith_type=Unsigned  n_bits=8  bin_pt=2  align_bp=on  dbl_ovrd=off  block_type=logical
      settings: xl_area=[1 0 0 1 0 0 0]  block_version=VER_STRING_GOES_HERE
  Register : xbsIndex_r4/Register  init=1  rst=off  en=off  dbl_ovrd=off  block_type=register
      settings: xl_area=[1 1 0 0 0 0 0]  block_version=VER_STRING_GOES_HERE
  Register1 : xbsIndex_r4/Register  init=0  rst=off  en=off  dbl_ovrd=off  block_type=register
      settings: xl_area=[1 1 0 0 0 0 0]  block_version=VER_STRING_GOES_HERE
  Relational : xbsIndex_r4/Relational  mode=a!=b  en=off  latency=0  dbl_ovrd=off  block_type=relational
      settings: xl_area=[1 0 0 1 0 0 0]  block_version=VER_STRING_GOES_HERE
  col lsb : xbsIndex_r4/Slice  nbits=1  boolean_output=off  mode=Lower Bit Location + Width  bit1=0  base1=MSB of Input  bit0=M-2  base0=LSB of Input  dbl_ovrd=off  block_type=slice
      settings: infoedit="Extracts a given range of bits from each input sample and presents it at the output.  The output type is ordinarily unsigned with binary point at zero, but can be Boolean when the slice is one bit wide.<P><P>Hardware notes: In hardware this block costs nothing."  block_version=VER_STRING_GOES_HERE
  col lsb1 : xbsIndex_r4/Slice  nbits=1  boolean_output=off  mode=Lower Bit Location + Width  bit1=0  base1=MSB of Input  bit0=M-2  base0=LSB of Input  dbl_ovrd=off  block_type=slice
      settings: infoedit="Extracts a given range of bits from each input sample and presents it at the output.  The output type is ordinarily unsigned with binary point at zero, but can be Boolean when the slice is one bit wide.<P><P>Hardware notes: In hardware this block costs nothing."  block_version=VER_STRING_GOES_HERE
  lsb : xbsIndex_r4/Slice  nbits=1  boolean_output=off  mode=Lower Bit Location + Width  bit1=0  base1=MSB of Input  bit0=0  base0=LSB of Input  dbl_ovrd=off  block_type=slice
      settings: infoedit="Extracts a given range of bits from each input sample and presents it at the output.  The output type is ordinarily unsigned with binary point at zero, but can be Boolean when the slice is one bit wide.<P><P>Hardware notes: In hardware this block costs nothing."  block_version=VER_STRING_GOES_HERE
  partial col : xbsIndex_r4/Slice  nbits=N-2  boolean_output=off  mode=Lower Bit Location + Width  bit1=0  base1=MSB of Input  bit0=0  base0=LSB of Input  dbl_ovrd=off  block_type=slice
      settings: infoedit="Extracts a given range of bits from each input sample and presents it at the output.  The output type is ordinarily unsigned with binary point at zero, but can be Boolean when the slice is one bit wide.<P><P>Hardware notes: In hardware this block costs nothing."  block_version=VER_STRING_GOES_HERE
  partial col1 : xbsIndex_r4/Slice  nbits=N-2  boolean_output=off  mode=Lower Bit Location + Width  bit1=0  base1=MSB of Input  bit0=0  base0=LSB of Input  dbl_ovrd=off  block_type=slice
      settings: infoedit="Extracts a given range of bits from each input sample and presents it at the output.  The output type is ordinarily unsigned with binary point at zero, but can be Boolean when the slice is one bit wide.<P><P>Hardware notes: In hardware this block costs nothing."  block_version=VER_STRING_GOES_HERE
  partial col2 : xbsIndex_r4/Slice  nbits=N-2  boolean_output=off  mode=Lower Bit Location + Width  bit1=0  base1=MSB of Input  bit0=0  base0=LSB of Input  dbl_ovrd=off  block_type=slice
      settings: infoedit="Extracts a given range of bits from each input sample and presents it at the output.  The output type is ordinarily unsigned with binary point at zero, but can be Boolean when the slice is one bit wide.<P><P>Hardware notes: In hardware this block costs nothing."  block_version=VER_STRING_GOES_HERE
  row : xbsIndex_r4/Slice  nbits=M-2  boolean_output=off  mode=Upper Bit Location + Width  bit1=0  base1=MSB of Input  bit0=N  base0=LSB of Input  dbl_ovrd=off  block_type=slice
      settings: infoedit="Extracts a given range of bits from each input sample and presents it at the output.  The output type is ordinarily unsigned with binary point at zero, but can be Boolean when the slice is one bit wide.<P><P>Hardware notes: In hardware this block costs nothing."  block_version=VER_STRING_GOES_HERE
  row1 : xbsIndex_r4/Slice  nbits=M-2  boolean_output=off  mode=Upper Bit Location + Width  bit1=0  base1=MSB of Input  bit0=N  base0=LSB of Input  dbl_ovrd=off  block_type=slice
      settings: infoedit="Extracts a given range of bits from each input sample and presents it at the output.  The output type is ordinarily unsigned with binary point at zero, but can be Boolean when the slice is one bit wide.<P><P>Hardware notes: In hardware this block costs nothing."  block_version=VER_STRING_GOES_HERE
  row2 : xbsIndex_r4/Slice  nbits=M-2  boolean_output=off  mode=Upper Bit Location + Width  bit1=0  base1=MSB of Input  bit0=N  base0=LSB of Input  dbl_ovrd=off  block_type=slice
      settings: infoedit="Extracts a given range of bits from each input sample and presents it at the output.  The output type is ordinarily unsigned with binary point at zero, but can be Boolean when the slice is one bit wide.<P><P>Hardware notes: In hardware this block costs nothing."  block_version=VER_STRING_GOES_HERE
  Bank 1 Read Addr : Outport  OutDataType=sfix(16)  OutScaling=2^0
  Bank 2 Read Addr : Outport  Port=2  OutDataType=sfix(16)  OutScaling=2^0
  H Filter W Addr : Outport  Port=3  OutDataType=sfix(16)  OutScaling=2^0
  L Filter W Addr : Outport  Port=4  OutDataType=sfix(16)  OutScaling=2^0
  Crossbar Switch : Outport  Port=5  OutDataType=sfix(16)  OutScaling=2^0
  sol : Outport  Port=6  OutDataType=sfix(16)  OutScaling=2^0
  eol : Outport  Port=7  OutDataType=sfix(16)  OutScaling=2^0
  wires:
  Logical/1 -> Crossbar Switch/1
  col lsb1/1 -> Logical/1
  Constant3/1 -> Concat7/1
  Constant1/1 -> Concat5/1
  partial col/1 -> Concat3/1, Concat1/1
  Constant4/1 -> Concat4/1
  Constant2/1 -> Concat2/1
  [long_count] -> row2/1, partial col2/1
  row2/1 -> Concat7/2
  Concat8/1 -> Bank 2 Read Addr/1
  Concat7/1 -> Concat8/2
  [long_count] -> row1/1, partial col1/1
  row1/1 -> Concat5/2
  Concat6/1 -> Bank 1 Read Addr/1
  Concat5/1 -> Concat6/2
  [long_count] -> col lsb/1
  col lsb/1 -> Relational/1, Register/1
  Relational/1 -> sol/1, Buffer6/1
  Buffer6/1 -> Register1/1
  [long_count] -> col lsb1/1, lsb/1
  lsb/1 -> Logical/2
  Register/1 -> Relational/2
  [long_count] -> row/1, partial col/1
  Concat3/1 -> Concat4/2
  Concat1/1 -> Concat2/2
  Concat2/1 -> H Filter W Addr/1
  Concat4/1 -> L Filter W Addr/1
  Register1/1 -> eol/1
  cnt/1 -> [long_count]
  Constant5/1 -> Concat9/1
  partial col2/1 -> Concat9/2
  Concat9/1 -> Concat8/1
  Constant6/1 -> Concat10/1
  partial col1/1 -> Concat10/2
  Concat10/1 -> Concat6/1
  Constant7/1 -> Concat11/1
  row/1 -> Concat11/2
  Concat11/1 -> Concat3/2, Concat1/2

== system sysgenDWT/Processor/Memory Controller/S-R FF ==
  note: 1-bit register used as Set-Reset Flip Flop.
  s : Inport  OutDataType=sfix(16)  OutScaling=2^0
  r : Inport  Port=2  OutDataType=sfix(16)  OutScaling=2^0
  Register2 : xbsIndex_r4/Register  init=0  rst=on  en=on  dbl_ovrd=off  block_type=register
      settings: xl_area=[1 1 0 0 0 0 0]  block_version=VER_STRING_GOES_HERE
  q : Outport  OutDataType=sfix(16)  OutScaling=2^0
  wires:
  s/1 -> Register2/1, Register2/3
  r/1 -> Register2/2
  Register2/1 -> q/1
